simulink library "halin"  (R2021b)
settings: Solver=VariableStepAuto  StartTime=0.0  StopTime=10.0  RelTol=1e-3
undefined symbols (not defined in the file): KHAL_CAN1ABM1E2E_flg, KHAL_CAN1ESC1E2E_flg, KHAL_CAN1ESC5E2E_flg, KHAL_CAN1ESC7E2E_flg, KHAL_CAN1FCM2E2E_flg, KHAL_CAN1FCM3E2E_flg, KHAL_CAN1FCM4E2E_flg, KHAL_CAN3BMS1E2E_flg, KHAL_CAN3BMS6E2E_flg, KHAL_CAN3CCU1E2E_flg, KHAL_CAN3CCU2E2E_flg, KHAL_CAN3MCUF1E2E_flg, KHAL_CAN3MCUR1E2E_flg, KHAL_CAN3Shifter1E2E_flg, TRUE
libraries: simulink x420, FVT_lib x149, hcu_lib x49
(part 8 of 14)

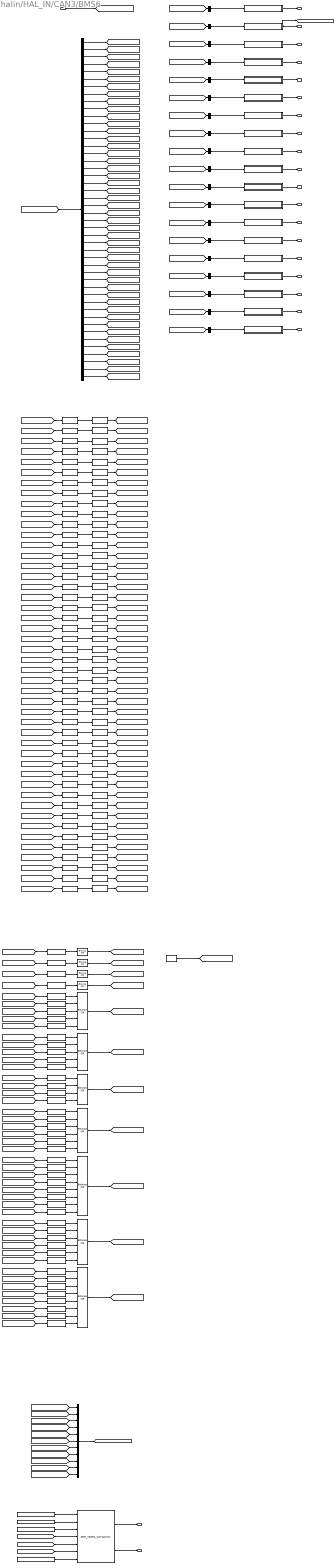
== system halin/HAL_IN/CAN3/BMS6 ==
  DT_CAN3_SG_BMS6 : Inport
  0x3b : Constant  Value=0x3b
  0xdb : Constant  Value=0xdb
  BMSChckSum : Subsystem
  BMSREADY : Subsystem
  BMSRolCnct : Subsystem
  BMSWarn1 : Subsystem
  BMSWarn2 : Subsystem
  BMSWarn3 : Subsystem
  BMSWarn4 : Subsystem
  BMSWarn5 : Subsystem
  BMSWarn6 : Subsystem
  BMSWarn7 : Subsystem
  BMSWarn8 : Subsystem
  BitwiseAND{,1..45} (46 alike) : simulink/Logic and Bit Operations/Bitwise Operator  logicop=AND  UseBitMask=on  BitMask=0xFF  BitMaskRealWorld=Stored Integer
  BitwiseOR{,1..3} (4 alike) : simulink/Logic and Bit Operations/Bitwise Operator  logicop=OR  UseBitMask=off  BitMask=bin2dec('11011001')  BitMaskRealWorld=Stored Integer
  BitwiseOR10 : simulink/Logic and Bit Operations/Bitwise Operator  logicop=OR  UseBitMask=off  NumInputPorts=8  BitMask=bin2dec('11011001')  BitMaskRealWorld=Stored Integer
  BitwiseOR4 : simulink/Logic and Bit Operations/Bitwise Operator  logicop=OR  UseBitMask=off  NumInputPorts=5  BitMask=bin2dec('11011001')  BitMaskRealWorld=Stored Integer
  BitwiseOR5 : simulink/Logic and Bit Operations/Bitwise Operator  logicop=OR  UseBitMask=off  NumInputPorts=5  BitMask=bin2dec('11011001')  BitMaskRealWorld=Stored Integer
  BitwiseOR6 : simulink/Logic and Bit Operations/Bitwise Operator  logicop=OR  UseBitMask=off  NumInputPorts=4  BitMask=bin2dec('11011001')  BitMaskRealWorld=Stored Integer
  BitwiseOR7 : simulink/Logic and Bit Operations/Bitwise Operator  logicop=OR  UseBitMask=off  NumInputPorts=6  BitMask=bin2dec('11011001')  BitMaskRealWorld=Stored Integer
  BitwiseOR8 : simulink/Logic and Bit Operations/Bitwise Operator  logicop=OR  UseBitMask=off  NumInputPorts=8  BitMask=bin2dec('11011001')  BitMaskRealWorld=Stored Integer
  BitwiseOR9 : simulink/Logic and Bit Operations/Bitwise Operator  logicop=OR  UseBitMask=off  NumInputPorts=6  BitMask=bin2dec('11011001')  BitMaskRealWorld=Stored Integer
  ChrgPlugSta : Subsystem
  DDM_CS&RC_Comparison : FVT_lib/hal/DDM_CS&RC_Comparison  MsgCycleTime=100
  Data Type Conversion{,1..45} (46 alike) : DataTypeConversion  OutDataTypeStr=uint8
  ExtChrgSta : Subsystem
  HVBContactorSta : Subsystem
  HVBHVILErr : Subsystem
  HVBPreheatPrecoolSta : Subsystem
  HVBattReady4Pre : Subsystem
  HVILSta : Subsystem
  KHAL_CAN3BMS6E2E_flg : Constant  Value=KHAL_CAN3BMS6E2E_flg
  LeftShift{,3,14,17,22,25,29,41,43,45} (10 alike) : ArithShift  BitShiftDirection=Left
  LeftShift{1,7,12,16,18,27,30..31} (8 alike) : ArithShift  BitShiftNumber=4  BitShiftDirection=Left
  LeftShift{10,24,35,42} (4 alike) : ArithShift  BitShiftNumber=7  BitShiftDirection=Left
  LeftShift{5,11,13,20,23,28,39} (7 alike) : ArithShift  BitShiftNumber=2  BitShiftDirection=Left
  LeftShift{9,15,19,32..34,36} (7 alike) : ArithShift  BitShiftNumber=6  BitShiftDirection=Left
  LeftShift{2,4,21,26,44} (5 alike) : ArithShift  BitShiftNumber=1  BitShiftDirection=Left
  LeftShift37 : ArithShift  BitShiftNumber=5  BitShiftDirection=Left
  LeftShift38 : ArithShift  BitShiftNumber=3  BitShiftDirection=Left
  LeftShift40 : ArithShift  BitShiftNumber=5  BitShiftDirection=Left
  LeftShift6 : ArithShift  BitShiftNumber=3  BitShiftDirection=Left
  LeftShift8 : ArithShift  BitShiftNumber=5  BitShiftDirection=Left
  MessageRollingCounter : FVT_lib/hal/MessageRollingCounter  CounterMAX=14  task_time_ms=5  msg_time_ms=100
  Mux : Mux  Inputs=11
  V2LSta : Subsystem
  bus_selector : BusSelector  OutputSignals=CAN3_BMSChckSum,CAN3_BMSRolCnct,CAN3_BMS_READY,CAN3_BMS_Warn_1,CAN3_BMS_Warn_2,CAN3_BMS_Warn_3,CAN3_BMS_Warn_4,CAN3_BMS_Warn_5,CAN3_BMS_Warn_6,CAN3_BMS_Warn_7,CAN3_BMS_Warn_8,CAN3_CellUnconsistErr,CAN3_ChrgInLockReq,CAN3_ChrgPlugSta,CAN3_DCChrgSysShockErr,CAN3_DisChrgPlugErr,CAN3_ExtChrgSta,CAN3_HVBCellOvrVoltErr,CAN3_HVBCellOvrVoltWarn,CAN3_HVBCellUdrVoltWarn,CAN3_HVBCellUnbalanErr,CAN3_HVBCellUndrVoltErr,CAN3_HVBChrgErr,CAN3_HVBContactorSta,CAN3_HVBHVILErr,CAN3_HVBOvrChrgCurrErr,CAN3_HVBOvrDchrgCurErr,CAN3_HVBOvrSOCErr,CAN3_HVBOvrTempErr,CAN3_HVBOvrTempWarn,CAN3_HVBOvrVoltErr,CAN3_HVBPrechrgSta,CAN3_HVBPreheatPrecoolSta,CAN3_HVBSOCJumpError,CAN3_HVBShrtChrgCurrErr,CAN3_HVBShrtDischrgCurrErr,CAN3_HVBTempDiffErr,CAN3_HVBUndrSOCErr,CAN3_HVBUndrTempErr,CAN3_HVBUndrTempWarn,CAN3_HVBUndrVoltErr,CAN3_HVBattReady4Pre,CAN3_HVILSta,CAN3_IsoDetSta,CAN3_SystemUncomErr,CAN3_V2LSta
  bus_selector1 : BusSelector  OutputSignals=CAN3_BMSChckSum
  bus_selector10 : BusSelector  OutputSignals=CAN3_BMS_Warn_7
  bus_selector11 : BusSelector  OutputSignals=CAN3_BMS_Warn_8
  bus_selector12 : BusSelector  OutputSignals=CAN3_ChrgPlugSta
  bus_selector13 : BusSelector  OutputSignals=CAN3_ExtChrgSta
  bus_selector14 : BusSelector  OutputSignals=CAN3_HVBContactorSta
  bus_selector15 : BusSelector  OutputSignals=CAN3_HVBHVILErr
  bus_selector16 : BusSelector  OutputSignals=CAN3_HVBPreheatPrecoolSta
  bus_selector17 : BusSelector  OutputSignals=CAN3_HVBattReady4Pre
  bus_selector18 : BusSelector  OutputSignals=CAN3_HVILSta
  bus_selector19 : BusSelector  OutputSignals=CAN3_V2LSta
  bus_selector2 : BusSelector  OutputSignals=CAN3_BMSRolCnct
  bus_selector3 : BusSelector  OutputSignals=CAN3_BMS_READY
  bus_selector4 : BusSelector  OutputSignals=CAN3_BMS_Warn_1
  bus_selector5 : BusSelector  OutputSignals=CAN3_BMS_Warn_2
  bus_selector6 : BusSelector  OutputSignals=CAN3_BMS_Warn_3
  bus_selector7 : BusSelector  OutputSignals=CAN3_BMS_Warn_4
  bus_selector8 : BusSelector  OutputSignals=CAN3_BMS_Warn_5
  bus_selector9 : BusSelector  OutputSignals=CAN3_BMS_Warn_6
  constant : Constant  Value=0x0  OutDataTypeStr=uint8
  VHAL_BMS6CSErr_flg : Outport
  VHAL_BMS6RCErr_flg : Outport  Port=2
  VHAL_BMSChckSum_enum : Outport  Port=3
  VHAL_BMSRolCnct_enum : Outport  Port=4
  VHAL_BMSREADY_flg : Outport  Port=5
  VHAL_BMSWarn1_flg : Outport  Port=6
  VHAL_BMSWarn2_flg : Outport  Port=7
  VHAL_BMSWarn3_flg : Outport  Port=8
  VHAL_BMSWarn4_flg : Outport  Port=9
  VHAL_BMSWarn5_flg : Outport  Port=10
  VHAL_BMSWarn6_flg : Outport  Port=11
  VHAL_BMSWarn7_flg : Outport  Port=12
  VHAL_BMSWarn8_flg : Outport  Port=13
  VHAL_ChrgPlugSta_enum : Outport  Port=14
  VHAL_ExtChrgSta_enum : Outport  Port=15
  VHAL_HVBContactorSta_flg : Outport  Port=16
  VHAL_HVBHVILErr_flg : Outport  Port=17
  VHAL_HVBPreheatPrecoolSta_enum : Outport  Port=18
  VHAL_HVBattReady4Pre_enum : Outport  Port=19
  VHAL_HVILSta_flg : Outport  Port=20
  VHAL_V2LSta_enum : Outport  Port=21
  wires:
  DT_CAN3_SG_BMS6/1 -> [DT_CAN3_SG_BMS6]
  [DT_CAN3_SG_BMS6] -> bus_selector/1
  bus_selector/1 -> [CAN3_BMSChckSum]  "<CAN3_BMSChckSum>"
  [CAN3_BMSChckSum] -> LeftShift/1
  LeftShift/1 -> BitwiseAND/1
  BitwiseAND/1 -> [Byte_0_CAN3_BMSChckSum]
  bus_selector/2 -> [CAN3_BMSRolCnct]  "<CAN3_BMSRolCnct>"
  [CAN3_BMSRolCnct] -> LeftShift1/1
  LeftShift1/1 -> BitwiseAND1/1
  BitwiseAND1/1 -> [Byte_1_CAN3_BMSRolCnct]
  bus_selector/3 -> [CAN3_BMS_READY]  "<CAN3_BMS_READY>"
  [CAN3_BMS_READY] -> LeftShift2/1
  LeftShift2/1 -> BitwiseAND2/1
  BitwiseAND2/1 -> [Byte_8_CAN3_BMS_READY]
  bus_selector/4 -> [CAN3_BMS_Warn_1]  "<CAN3_BMS_Warn_1>"
  [CAN3_BMS_Warn_1] -> LeftShift3/1
  LeftShift3/1 -> BitwiseAND3/1
  BitwiseAND3/1 -> [Byte_11_CAN3_BMS_Warn_1]
  bus_selector/5 -> [CAN3_BMS_Warn_2]  "<CAN3_BMS_Warn_2>"
  [CAN3_BMS_Warn_2] -> LeftShift4/1
  LeftShift4/1 -> BitwiseAND4/1
  BitwiseAND4/1 -> [Byte_11_CAN3_BMS_Warn_2]
  bus_selector/6 -> [CAN3_BMS_Warn_3]  "<CAN3_BMS_Warn_3>"
  [CAN3_BMS_Warn_3] -> LeftShift5/1
  LeftShift5/1 -> BitwiseAND5/1
  BitwiseAND5/1 -> [Byte_11_CAN3_BMS_Warn_3]
  bus_selector/7 -> [CAN3_BMS_Warn_4]  "<CAN3_BMS_Warn_4>"
  [CAN3_BMS_Warn_4] -> LeftShift6/1
  LeftShift6/1 -> BitwiseAND6/1
  BitwiseAND6/1 -> [Byte_11_CAN3_BMS_Warn_4]
  bus_selector/8 -> [CAN3_BMS_Warn_5]  "<CAN3_BMS_Warn_5>"
  [CAN3_BMS_Warn_5] -> LeftShift7/1
  LeftShift7/1 -> BitwiseAND7/1
  BitwiseAND7/1 -> [Byte_11_CAN3_BMS_Warn_5]
  bus_selector/9 -> [CAN3_BMS_Warn_6]  "<CAN3_BMS_Warn_6>"
  [CAN3_BMS_Warn_6] -> LeftShift8/1
  LeftShift8/1 -> BitwiseAND8/1
  BitwiseAND8/1 -> [Byte_11_CAN3_BMS_Warn_6]
  bus_selector/10 -> [CAN3_BMS_Warn_7]  "<CAN3_BMS_Warn_7>"
  [CAN3_BMS_Warn_7] -> LeftShift9/1
  LeftShift9/1 -> BitwiseAND9/1
  BitwiseAND9/1 -> [Byte_11_CAN3_BMS_Warn_7]
  bus_selector/11 -> [CAN3_BMS_Warn_8]  "<CAN3_BMS_Warn_8>"
  [CAN3_BMS_Warn_8] -> LeftShift10/1
  LeftShift10/1 -> BitwiseAND10/1
  BitwiseAND10/1 -> [Byte_11_CAN3_BMS_Warn_8]
  bus_selector/12 -> [CAN3_CellUnconsistErr]  "<CAN3_CellUnconsistErr>"
  [CAN3_CellUnconsistErr] -> LeftShift11/1
  LeftShift11/1 -> BitwiseAND11/1
  BitwiseAND11/1 -> [Byte_6_CAN3_CellUnconsistErr]
  bus_selector/13 -> [CAN3_ChrgInLockReq]  "<CAN3_ChrgInLockReq>"
  [CAN3_ChrgInLockReq] -> LeftShift12/1
  LeftShift12/1 -> BitwiseAND12/1
  BitwiseAND12/1 -> [Byte_5_CAN3_ChrgInLockReq]
  bus_selector/14 -> [CAN3_ChrgPlugSta]  "<CAN3_ChrgPlugSta>"
  [CAN3_ChrgPlugSta] -> LeftShift13/1
  LeftShift13/1 -> BitwiseAND13/1
  BitwiseAND13/1 -> [Byte_7_CAN3_ChrgPlugSta]
  bus_selector/15 -> [CAN3_DCChrgSysShockErr]  "<CAN3_DCChrgSysShockErr>"
  [CAN3_DCChrgSysShockErr] -> LeftShift14/1
  LeftShift14/1 -> BitwiseAND14/1
  BitwiseAND14/1 -> [Byte_8_CAN3_DCChrgSysShockErr]
  bus_selector/16 -> [CAN3_DisChrgPlugErr]  "<CAN3_DisChrgPlugErr>"
  [CAN3_DisChrgPlugErr] -> LeftShift15/1
  LeftShift15/1 -> BitwiseAND15/1
  BitwiseAND15/1 -> [Byte_5_CAN3_DisChrgPlugErr]
  bus_selector/17 -> [CAN3_ExtChrgSta]  "<CAN3_ExtChrgSta>"
  [CAN3_ExtChrgSta] -> LeftShift16/1
  LeftShift16/1 -> BitwiseAND16/1
  BitwiseAND16/1 -> [Byte_7_CAN3_ExtChrgSta]
  bus_selector/18 -> [CAN3_HVBCellOvrVoltErr]  "<CAN3_HVBCellOvrVoltErr>"
  [CAN3_HVBCellOvrVoltErr] -> LeftShift17/1
  LeftShift17/1 -> BitwiseAND17/1
  BitwiseAND17/1 -> [Byte_5_CAN3_HVBCellOvrVoltErr]
  bus_selector/19 -> [CAN3_HVBCellOvrVoltWarn]  "<CAN3_HVBCellOvrVoltWarn>"
  [CAN3_HVBCellOvrVoltWarn] -> LeftShift18/1
  LeftShift18/1 -> BitwiseAND18/1
  BitwiseAND18/1 -> [Byte_6_CAN3_HVBCellOvrVoltWarn]
  bus_selector/20 -> [CAN3_HVBCellUdrVoltWarn]  "<CAN3_HVBCellUdrVoltWarn>"
  [CAN3_HVBCellUdrVoltWarn] -> LeftShift19/1
  LeftShift19/1 -> BitwiseAND19/1
  BitwiseAND19/1 -> [Byte_6_CAN3_HVBCellUdrVoltWarn]
  bus_selector/21 -> [CAN3_HVBCellUnbalanErr]  "<CAN3_HVBCellUnbalanErr>"
  [CAN3_HVBCellUnbalanErr] -> LeftShift20/1
  LeftShift20/1 -> BitwiseAND20/1
  BitwiseAND20/1 -> [Byte_5_CAN3_HVBCellUnbalanErr]
  bus_selector/22 -> [CAN3_HVBCellUndrVoltErr]  "<CAN3_HVBCellUndrVoltErr>"
  [CAN3_HVBCellUndrVoltErr] -> LeftShift21/1
  LeftShift21/1 -> BitwiseAND21/1
  BitwiseAND21/1 -> [Byte_5_CAN3_HVBCellUndrVoltErr]
  bus_selector/23 -> [CAN3_HVBChrgErr]  "<CAN3_HVBChrgErr>"
  [CAN3_HVBChrgErr] -> LeftShift22/1
  LeftShift22/1 -> BitwiseAND22/1
  BitwiseAND22/1 -> [Byte_4_CAN3_HVBChrgErr]
  bus_selector/24 -> [CAN3_HVBContactorSta]  "<CAN3_HVBContactorSta>"
  [CAN3_HVBContactorSta] -> LeftShift23/1
  LeftShift23/1 -> BitwiseAND23/1
  BitwiseAND23/1 -> [Byte_8_CAN3_HVBContactorSta]
  bus_selector/25 -> [CAN3_HVBHVILErr]  "<CAN3_HVBHVILErr>"
  [CAN3_HVBHVILErr] -> LeftShift24/1
  LeftShift24/1 -> BitwiseAND24/1
  BitwiseAND24/1 -> [Byte_9_CAN3_HVBHVILErr]
  bus_selector/26 -> [CAN3_HVBOvrChrgCurrErr]  "<CAN3_HVBOvrChrgCurrErr>"
  [CAN3_HVBOvrChrgCurrErr] -> LeftShift25/1
  LeftShift25/1 -> BitwiseAND25/1
  BitwiseAND25/1 -> [Byte_9_CAN3_HVBOvrChrgCurrErr]
  bus_selector/27 -> [CAN3_HVBOvrDchrgCurErr]  "<CAN3_HVBOvrDchrgCurErr>"
  [CAN3_HVBOvrDchrgCurErr] -> LeftShift26/1
  LeftShift26/1 -> BitwiseAND26/1
  BitwiseAND26/1 -> [Byte_9_CAN3_HVBOvrDchrgCurErr]
  bus_selector/28 -> [CAN3_HVBOvrSOCErr]  "<CAN3_HVBOvrSOCErr>"
  [CAN3_HVBOvrSOCErr] -> LeftShift27/1
  LeftShift27/1 -> BitwiseAND27/1
  BitwiseAND27/1 -> [Byte_9_CAN3_HVBOvrSOCErr]
  bus_selector/29 -> [CAN3_HVBOvrTempErr]  "<CAN3_HVBOvrTempErr>"
  [CAN3_HVBOvrTempErr] -> LeftShift28/1
  LeftShift28/1 -> BitwiseAND28/1
  BitwiseAND28/1 -> [Byte_9_CAN3_HVBOvrTempErr]
  bus_selector/30 -> [CAN3_HVBOvrTempWarn]  "<CAN3_HVBOvrTempWarn>"
  [CAN3_HVBOvrTempWarn] -> LeftShift29/1
  LeftShift29/1 -> BitwiseAND29/1
  BitwiseAND29/1 -> [Byte_10_CAN3_HVBOvrTempWarn]
  bus_selector/31 -> [CAN3_HVBOvrVoltErr]  "<CAN3_HVBOvrVoltErr>"
  [CAN3_HVBOvrVoltErr] -> LeftShift30/1
  LeftShift30/1 -> BitwiseAND30/1
  BitwiseAND30/1 -> [Byte_10_CAN3_HVBOvrVoltErr]
  bus_selector/32 -> [CAN3_HVBPrechrgSta]  "<CAN3_HVBPrechrgSta>"
  [CAN3_HVBPrechrgSta] -> LeftShift31/1
  LeftShift31/1 -> BitwiseAND31/1
  BitwiseAND31/1 -> [Byte_8_CAN3_HVBPrechrgSta]
  bus_selector/33 -> [CAN3_HVBPreheatPrecoolSta]  "<CAN3_HVBPreheatPrecoolSta>"
  [CAN3_HVBPreheatPrecoolSta] -> LeftShift32/1
  LeftShift32/1 -> BitwiseAND32/1
  BitwiseAND32/1 -> [Byte_7_CAN3_HVBPreheatPrecoolSta]
  bus_selector/34 -> [CAN3_HVBSOCJumpError]  "<CAN3_HVBSOCJumpError>"
  [CAN3_HVBSOCJumpError] -> LeftShift33/1
  LeftShift33/1 -> BitwiseAND33/1
  BitwiseAND33/1 -> [Byte_9_CAN3_HVBSOCJumpError]
  bus_selector/35 -> [CAN3_HVBShrtChrgCurrErr]  "<CAN3_HVBShrtChrgCurrErr>"
  [CAN3_HVBShrtChrgCurrErr] -> LeftShift34/1
  LeftShift34/1 -> BitwiseAND34/1
  BitwiseAND34/1 -> [Byte_10_CAN3_HVBShrtChrgCurrErr]
  bus_selector/36 -> [CAN3_HVBShrtDischrgCurrErr]  "<CAN3_HVBShrtDischrgCurrErr>"
  [CAN3_HVBShrtDischrgCurrErr] -> LeftShift35/1
  LeftShift35/1 -> BitwiseAND35/1
  BitwiseAND35/1 -> [Byte_10_CAN3_HVBShrtDischrgCurrErr]
  bus_selector/37 -> [CAN3_HVBTempDiffErr]  "<CAN3_HVBTempDiffErr>"
  [CAN3_HVBTempDiffErr] -> LeftShift36/1
  LeftShift36/1 -> BitwiseAND36/1
  BitwiseAND36/1 -> [Byte_8_CAN3_HVBTempDiffErr]
  bus_selector/38 -> [CAN3_HVBUndrSOCErr]  "<CAN3_HVBUndrSOCErr>"
  [CAN3_HVBUndrSOCErr] -> LeftShift37/1
  LeftShift37/1 -> BitwiseAND37/1
  BitwiseAND37/1 -> [Byte_9_CAN3_HVBUndrSOCErr]
  bus_selector/39 -> [CAN3_HVBUndrTempErr]  "<CAN3_HVBUndrTempErr>"
  [CAN3_HVBUndrTempErr] -> LeftShift38/1
  LeftShift38/1 -> BitwiseAND38/1
  BitwiseAND38/1 -> [Byte_9_CAN3_HVBUndrTempErr]
  bus_selector/40 -> [CAN3_HVBUndrTempWarn]  "<CAN3_HVBUndrTempWarn>"
  [CAN3_HVBUndrTempWarn] -> LeftShift39/1
  LeftShift39/1 -> BitwiseAND39/1
  BitwiseAND39/1 -> [Byte_10_CAN3_HVBUndrTempWarn]
  bus_selector/41 -> [CAN3_HVBUndrVoltErr]  "<CAN3_HVBUndrVoltErr>"
  [CAN3_HVBUndrVoltErr] -> LeftShift40/1
  LeftShift40/1 -> BitwiseAND40/1
  BitwiseAND40/1 -> [Byte_10_CAN3_HVBUndrVoltErr]
  bus_selector/42 -> [CAN3_HVBattReady4Pre]  "<CAN3_HVBattReady4Pre>"
  [CAN3_HVBattReady4Pre] -> LeftShift41/1
  LeftShift41/1 -> BitwiseAND41/1
  BitwiseAND41/1 -> [Byte_7_CAN3_HVBattReady4Pre]
  bus_selector/43 -> [CAN3_HVILSta]  "<CAN3_HVILSta>"
  [CAN3_HVILSta] -> LeftShift42/1
  LeftShift42/1 -> BitwiseAND42/1
  BitwiseAND42/1 -> [Byte_8_CAN3_HVILSta]
  bus_selector/44 -> [CAN3_IsoDetSta]  "<CAN3_IsoDetSta>"
  [CAN3_IsoDetSta] -> LeftShift43/1
  LeftShift43/1 -> BitwiseAND43/1
  BitwiseAND43/1 -> [Byte_6_CAN3_IsoDetSta]
  bus_selector/45 -> [CAN3_SystemUncomErr]  "<CAN3_SystemUncomErr>"
  [CAN3_SystemUncomErr] -> LeftShift44/1
  LeftShift44/1 -> BitwiseAND44/1
  BitwiseAND44/1 -> [Byte_6_CAN3_SystemUncomErr]
  bus_selector/46 -> [CAN3_V2LSta]  "<CAN3_V2LSta>"
  [CAN3_V2LSta] -> LeftShift45/1
  LeftShift45/1 -> BitwiseAND45/1
  BitwiseAND45/1 -> [Byte_3_CAN3_V2LSta]
  Data Type Conversion/1 -> BitwiseOR/1
  [Byte_0_CAN3_BMSChckSum] -> Data Type Conversion/1
  BitwiseOR/1 -> [Byte_0]
  Data Type Conversion1/1 -> BitwiseOR1/1
  [Byte_1_CAN3_BMSRolCnct] -> Data Type Conversion1/1
  BitwiseOR1/1 -> [Byte_1]
  constant/1 -> [Byte_2]
  Data Type Conversion2/1 -> BitwiseOR2/1
  [Byte_3_CAN3_V2LSta] -> Data Type Conversion2/1
  BitwiseOR2/1 -> [Byte_3]
  Data Type Conversion3/1 -> BitwiseOR3/1
  [Byte_4_CAN3_HVBChrgErr] -> Data Type Conversion3/1
  BitwiseOR3/1 -> [Byte_4]
  Data Type Conversion4/1 -> BitwiseOR4/1
  [Byte_5_CAN3_ChrgInLockReq] -> Data Type Conversion4/1
  Data Type Conversion5/1 -> BitwiseOR4/2
  [Byte_5_CAN3_DisChrgPlugErr] -> Data Type Conversion5/1
  Data Type Conversion6/1 -> BitwiseOR4/3
  [Byte_5_CAN3_HVBCellOvrVoltErr] -> Data Type Conversion6/1
  Data Type Conversion7/1 -> BitwiseOR4/4
  [Byte_5_CAN3_HVBCellUnbalanErr] -> Data Type Conversion7/1
  Data Type Conversion8/1 -> BitwiseOR4/5
  [Byte_5_CAN3_HVBCellUndrVoltErr] -> Data Type Conversion8/1
  BitwiseOR4/1 -> [Byte_5]
  Data Type Conversion9/1 -> BitwiseOR5/1
  [Byte_6_CAN3_CellUnconsistErr] -> Data Type Conversion9/1
  Data Type Conversion10/1 -> BitwiseOR5/2
  [Byte_6_CAN3_HVBCellOvrVoltWarn] -> Data Type Conversion10/1
  Data Type Conversion11/1 -> BitwiseOR5/3
  [Byte_6_CAN3_HVBCellUdrVoltWarn] -> Data Type Conversion11/1
  Data Type Conversion12/1 -> BitwiseOR5/4
  [Byte_6_CAN3_IsoDetSta] -> Data Type Conversion12/1
  Data Type Conversion13/1 -> BitwiseOR5/5
  [Byte_6_CAN3_SystemUncomErr] -> Data Type Conversion13/1
  BitwiseOR5/1 -> [Byte_6]
  Data Type Conversion14/1 -> BitwiseOR6/1
  [Byte_7_CAN3_ChrgPlugSta] -> Data Type Conversion14/1
  Data Type Conversion15/1 -> BitwiseOR6/2
  [Byte_7_CAN3_ExtChrgSta] -> Data Type Conversion15/1
  Data Type Conversion16/1 -> BitwiseOR6/3
  [Byte_7_CAN3_HVBPreheatPrecoolSta] -> Data Type Conversion16/1
  Data Type Conversion17/1 -> BitwiseOR6/4
  [Byte_7_CAN3_HVBattReady4Pre] -> Data Type Conversion17/1
  BitwiseOR6/1 -> [Byte_7]
  Data Type Conversion18/1 -> BitwiseOR7/1
  [Byte_8_CAN3_BMS_READY] -> Data Type Conversion18/1
  Data Type Conversion19/1 -> BitwiseOR7/2
  [Byte_8_CAN3_DCChrgSysShockErr] -> Data Type Conversion19/1
  Data Type Conversion20/1 -> BitwiseOR7/3
  [Byte_8_CAN3_HVBContactorSta] -> Data Type Conversion20/1
  Data Type Conversion21/1 -> BitwiseOR7/4
  [Byte_8_CAN3_HVBPrechrgSta] -> Data Type Conversion21/1
  Data Type Conversion22/1 -> BitwiseOR7/5
  [Byte_8_CAN3_HVBTempDiffErr] -> Data Type Conversion22/1
  Data Type Conversion23/1 -> BitwiseOR7/6
  [Byte_8_CAN3_HVILSta] -> Data Type Conversion23/1
  BitwiseOR7/1 -> [Byte_8]
  Data Type Conversion24/1 -> BitwiseOR8/1
  [Byte_9_CAN3_HVBHVILErr] -> Data Type Conversion24/1
  Data Type Conversion25/1 -> BitwiseOR8/2
  [Byte_9_CAN3_HVBOvrChrgCurrErr] -> Data Type Conversion25/1
  Data Type Conversion26/1 -> BitwiseOR8/3
  [Byte_9_CAN3_HVBOvrDchrgCurErr] -> Data Type Conversion26/1
  Data Type Conversion27/1 -> BitwiseOR8/4
  [Byte_9_CAN3_HVBOvrSOCErr] -> Data Type Conversion27/1
  Data Type Conversion28/1 -> BitwiseOR8/5
  [Byte_9_CAN3_HVBOvrTempErr] -> Data Type Conversion28/1
  Data Type Conversion29/1 -> BitwiseOR8/6
  [Byte_9_CAN3_HVBSOCJumpError] -> Data Type Conversion29/1
  Data Type Conversion30/1 -> BitwiseOR8/7
  [Byte_9_CAN3_HVBUndrSOCErr] -> Data Type Conversion30/1
  Data Type Conversion31/1 -> BitwiseOR8/8
  [Byte_9_CAN3_HVBUndrTempErr] -> Data Type Conversion31/1
  BitwiseOR8/1 -> [Byte_9]
  Data Type Conversion32/1 -> BitwiseOR9/1
  [Byte_10_CAN3_HVBOvrTempWarn] -> Data Type Conversion32/1
  Data Type Conversion33/1 -> BitwiseOR9/2
  [Byte_10_CAN3_HVBOvrVoltErr] -> Data Type Conversion33/1
  Data Type Conversion34/1 -> BitwiseOR9/3
  [Byte_10_CAN3_HVBShrtChrgCurrErr] -> Data Type Conversion34/1
  Data Type Conversion35/1 -> BitwiseOR9/4
  [Byte_10_CAN3_HVBShrtDischrgCurrErr] -> Data Type Conversion35/1
  Data Type Conversion36/1 -> BitwiseOR9/5
  [Byte_10_CAN3_HVBUndrTempWarn] -> Data Type Conversion36/1
  Data Type Conversion37/1 -> BitwiseOR9/6
  [Byte_10_CAN3_HVBUndrVoltErr] -> Data Type Conversion37/1
  BitwiseOR9/1 -> [Byte_10]
  Data Type Conversion38/1 -> BitwiseOR10/1
  [Byte_11_CAN3_BMS_Warn_1] -> Data Type Conversion38/1
  Data Type Conversion39/1 -> BitwiseOR10/2
  [Byte_11_CAN3_BMS_Warn_2] -> Data Type Conversion39/1
  Data Type Conversion40/1 -> BitwiseOR10/3
  [Byte_11_CAN3_BMS_Warn_3] -> Data Type Conversion40/1
  Data Type Conversion41/1 -> BitwiseOR10/4
  [Byte_11_CAN3_BMS_Warn_4] -> Data Type Conversion41/1
  Data Type Conversion42/1 -> BitwiseOR10/5
  [Byte_11_CAN3_BMS_Warn_5] -> Data Type Conversion42/1
  Data Type Conversion43/1 -> BitwiseOR10/6
  [Byte_11_CAN3_BMS_Warn_6] -> Data Type Conversion43/1
  Data Type Conversion44/1 -> BitwiseOR10/7
  [Byte_11_CAN3_BMS_Warn_7] -> Data Type Conversion44/1
  Data Type Conversion45/1 -> BitwiseOR10/8
  [Byte_11_CAN3_BMS_Warn_8] -> Data Type Conversion45/1
  BitwiseOR10/1 -> [Byte_11]
  [Byte_1] -> Mux/1
  [Byte_2] -> Mux/2
  [Byte_3] -> Mux/3
  [Byte_4] -> Mux/4
  [Byte_5] -> Mux/5
  [Byte_6] -> Mux/6
  [Byte_7] -> Mux/7
  [Byte_8] -> Mux/8
  [Byte_9] -> Mux/9
  [Byte_10] -> Mux/10
  [Byte_11] -> Mux/11
  Mux/1 -> [VHAL_CAN3BMS6noCS_raw]
  KHAL_CAN3BMS6E2E_flg/1 -> DDM_CS&RC_Comparison/1
  0x3b/1 -> DDM_CS&RC_Comparison/2
  0xdb/1 -> DDM_CS&RC_Comparison/3
  [VHAL_CAN3BMS6noCS_raw] -> DDM_CS&RC_Comparison/4
  [Byte_0] -> DDM_CS&RC_Comparison/5
  [RC_ECU] -> DDM_CS&RC_Comparison/6
  MessageRollingCounter/1 -> DDM_CS&RC_Comparison/7
  DDM_CS&RC_Comparison/1 -> VHAL_BMS6CSErr_flg/1
  DDM_CS&RC_Comparison/2 -> VHAL_BMS6RCErr_flg/1
  [DT_CAN3_SG_BMS6] -> bus_selector1/1
  bus_selector1/1 -> BMSChckSum/1(BMSChckSum)  "<CAN3_BMSChckSum>"
  BMSChckSum/1(VHAL_BMSChckSum_enum) -> VHAL_BMSChckSum_enum/1
  [DT_CAN3_SG_BMS6] -> bus_selector2/1
  bus_selector2/1 -> BMSRolCnct/1(BMSRolCnct)  "<CAN3_BMSRolCnct>"
  BMSRolCnct/1(VHAL_BMSRolCnct_enum) -> VHAL_BMSRolCnct_enum/1, [RC_ECU]
  [DT_CAN3_SG_BMS6] -> bus_selector3/1
  bus_selector3/1 -> BMSREADY/1(BMS_READY)  "<CAN3_BMS_READY>"
  BMSREADY/1(VHAL_BMSREADY_flg) -> VHAL_BMSREADY_flg/1
  [DT_CAN3_SG_BMS6] -> bus_selector4/1
  bus_selector4/1 -> BMSWarn1/1(BMS_Warn_1)  "<CAN3_BMS_Warn_1>"
  BMSWarn1/1(VHAL_BMSWarn1_flg) -> VHAL_BMSWarn1_flg/1
  [DT_CAN3_SG_BMS6] -> bus_selector5/1
  bus_selector5/1 -> BMSWarn2/1(BMS_Warn_2)  "<CAN3_BMS_Warn_2>"
  BMSWarn2/1(VHAL_BMSWarn2_flg) -> VHAL_BMSWarn2_flg/1
  [DT_CAN3_SG_BMS6] -> bus_selector6/1
  bus_selector6/1 -> BMSWarn3/1(BMS_Warn_3)  "<CAN3_BMS_Warn_3>"
  BMSWarn3/1(VHAL_BMSWarn3_flg) -> VHAL_BMSWarn3_flg/1
  [DT_CAN3_SG_BMS6] -> bus_selector7/1
  bus_selector7/1 -> BMSWarn4/1(BMS_Warn_4)  "<CAN3_BMS_Warn_4>"
  BMSWarn4/1(VHAL_BMSWarn4_flg) -> VHAL_BMSWarn4_flg/1
  [DT_CAN3_SG_BMS6] -> bus_selector8/1
  bus_selector8/1 -> BMSWarn5/1(BMS_Warn_5)  "<CAN3_BMS_Warn_5>"
  BMSWarn5/1(VHAL_BMSWarn5_flg) -> VHAL_BMSWarn5_flg/1
  [DT_CAN3_SG_BMS6] -> bus_selector9/1
  bus_selector9/1 -> BMSWarn6/1(BMS_Warn_6)  "<CAN3_BMS_Warn_6>"
  BMSWarn6/1(VHAL_BMSWarn6_flg) -> VHAL_BMSWarn6_flg/1
  [DT_CAN3_SG_BMS6] -> bus_selector10/1
  bus_selector10/1 -> BMSWarn7/1(BMS_Warn_7)  "<CAN3_BMS_Warn_7>"
  BMSWarn7/1(VHAL_BMSWarn7_flg) -> VHAL_BMSWarn7_flg/1
  [DT_CAN3_SG_BMS6] -> bus_selector11/1
  bus_selector11/1 -> BMSWarn8/1(BMS_Warn_8)  "<CAN3_BMS_Warn_8>"
  BMSWarn8/1(VHAL_BMSWarn8_flg) -> VHAL_BMSWarn8_flg/1
  [DT_CAN3_SG_BMS6] -> bus_selector12/1
  bus_selector12/1 -> ChrgPlugSta/1(ChrgPlugSta)  "<CAN3_ChrgPlugSta>"
  ChrgPlugSta/1(VHAL_ChrgPlugSta_enum) -> VHAL_ChrgPlugSta_enum/1
  [DT_CAN3_SG_BMS6] -> bus_selector13/1
  bus_selector13/1 -> ExtChrgSta/1(ExtChrgSta)  "<CAN3_ExtChrgSta>"
  ExtChrgSta/1(VHAL_ExtChrgSta_enum) -> VHAL_ExtChrgSta_enum/1
  [DT_CAN3_SG_BMS6] -> bus_selector14/1
  bus_selector14/1 -> HVBContactorSta/1(HVBContactorSta)  "<CAN3_HVBContactorSta>"
  HVBContactorSta/1(VHAL_HVBContactorSta_flg) -> VHAL_HVBContactorSta_flg/1
  [DT_CAN3_SG_BMS6] -> bus_selector15/1
  bus_selector15/1 -> HVBHVILErr/1(HVBHVILErr)  "<CAN3_HVBHVILErr>"
  HVBHVILErr/1(VHAL_HVBHVILErr_flg) -> VHAL_HVBHVILErr_flg/1
  [DT_CAN3_SG_BMS6] -> bus_selector16/1
  bus_selector16/1 -> HVBPreheatPrecoolSta/1(HVBPreheatPrecoolSta)  "<CAN3_HVBPreheatPrecoolSta>"
  HVBPreheatPrecoolSta/1(VHAL_HVBPreheatPrecoolSta_enum) -> VHAL_HVBPreheatPrecoolSta_enum/1
  [DT_CAN3_SG_BMS6] -> bus_selector17/1
  bus_selector17/1 -> HVBattReady4Pre/1(HVBattReady4Pre)  "<CAN3_HVBattReady4Pre>"
  HVBattReady4Pre/1(VHAL_HVBattReady4Pre_enum) -> VHAL_HVBattReady4Pre_enum/1
  [DT_CAN3_SG_BMS6] -> bus_selector18/1
  bus_selector18/1 -> HVILSta/1(HVILSta)  "<CAN3_HVILSta>"
  HVILSta/1(VHAL_HVILSta_flg) -> VHAL_HVILSta_flg/1
  [DT_CAN3_SG_BMS6] -> bus_selector19/1
  bus_selector19/1 -> V2LSta/1(V2LSta)  "<CAN3_V2LSta>"
  V2LSta/1(VHAL_V2LSta_enum) -> VHAL_V2LSta_enum/1

== system halin/HAL_IN/CAN3/BMS7 ==
  DT_CAN3_SG_BMS7 : Inport
  HVBattErr : Subsystem
  bus_selector : BusSelector  OutputSignals=CAN3_HVBattErr
  VHAL_HVBattErr_flg : Outport
  wires:
  DT_CAN3_SG_BMS7/1 -> [DT_CAN3_SG_BMS7]
  [DT_CAN3_SG_BMS7] -> bus_selector/1
  bus_selector/1 -> HVBattErr/1(HVBattErr)  "<CAN3_HVBattErr>"
  HVBattErr/1(VHAL_HVBattErr_flg) -> VHAL_HVBattErr_flg/1

== system halin/HAL_IN/CAN3/CCU1 ==
  DT_CAN3_SG_CCU1 : Inport
  0x35 : Constant  Value=0x35
  0xeb : Constant  Value=0xeb
  BitwiseAND{,1..11} (12 alike) : simulink/Logic and Bit Operations/Bitwise Operator  logicop=AND  UseBitMask=on  BitMask=0xFF  BitMaskRealWorld=Stored Integer
  BitwiseOR{,2,4..7} (6 alike) : simulink/Logic and Bit Operations/Bitwise Operator  logicop=OR  UseBitMask=off  BitMask=bin2dec('11011001')  BitMaskRealWorld=Stored Integer
  BitwiseOR1 : simulink/Logic and Bit Operations/Bitwise Operator  logicop=OR  UseBitMask=off  NumInputPorts=3  BitMask=bin2dec('11011001')  BitMaskRealWorld=Stored Integer
  BitwiseOR3 : simulink/Logic and Bit Operations/Bitwise Operator  logicop=OR  UseBitMask=off  NumInputPorts=3  BitMask=bin2dec('11011001')  BitMaskRealWorld=Stored Integer
  CSCCU1 : Subsystem
  DCDCAuxVolt : Subsystem
  DCDCInVoltInf : Subsystem
  DCDCPreCompleted : Subsystem
  DDM_CS&RC_Comparison : FVT_lib/hal/DDM_CS&RC_Comparison  MsgCycleTime=10
  Data Type Conversion{,1..11} (12 alike) : DataTypeConversion  OutDataTypeStr=uint8
  KHAL_CAN3CCU1E2E_flg : Constant  Value=KHAL_CAN3CCU1E2E_flg
  LeftShift : ArithShift  BitShiftDirection=Left
  LeftShift1 : ArithShift  BitShiftDirection=Left
  LeftShift2 : ArithShift  BitShiftNumber=4  BitShiftDirection=Left
  LeftShift3 : ArithShift  BitShiftNumber=6  BitShiftDirection=Left
  LeftShift4 : ArithShift  BitShiftNumber=2  BitShiftDirection=Left
  LeftShift5 : ArithShift  BitShiftDirection=Left
  MessageRollingCounter : FVT_lib/hal/MessageRollingCounter  CounterMAX=14  task_time_ms=5  msg_time_ms=10
  Mux : Mux  Inputs=7
  OBCDCCurrInf : Subsystem
  OBCDCVoltInf : Subsystem
  OBCPreCompleted : Subsystem
  OBCWakeup4Plugin : Subsystem
  RCCCU1 : Subsystem
  RightShift : ArithShift  BitShiftNumber=8
  RightShift1 : ArithShift
  RightShift2 : ArithShift  BitShiftNumber=8
  RightShift3 : ArithShift
  RightShift4 : ArithShift  BitShiftNumber=4
  RightShift5 : ArithShift  BitShiftNumber=-4
  bus_selector : BusSelector  OutputSignals=CAN3_CS_CCU1,CAN3_DCDCAuxVolt,CAN3_DCDCInVoltInf,CAN3_DCDCPreCompleted,CAN3_OBCDCCurrInf,CAN3_OBCDCVoltInf,CAN3_OBCPreCompleted,CAN3_OBCWakeup4Plugin,CAN3_RC_CCU1
  bus_selector1 : BusSelector  OutputSignals=CAN3_CS_CCU1
  bus_selector2 : BusSelector  OutputSignals=CAN3_DCDCAuxVolt
  bus_selector3 : BusSelector  OutputSignals=CAN3_DCDCInVoltInf
  bus_selector4 : BusSelector  OutputSignals=CAN3_DCDCPreCompleted
  bus_selector5 : BusSelector  OutputSignals=CAN3_OBCDCCurrInf
  bus_selector6 : BusSelector  OutputSignals=CAN3_OBCDCVoltInf
  bus_selector7 : BusSelector  OutputSignals=CAN3_OBCPreCompleted
  bus_selector8 : BusSelector  OutputSignals=CAN3_OBCWakeup4Plugin
  bus_selector9 : BusSelector  OutputSignals=CAN3_RC_CCU1
  VHAL_CCU1CSErr_flg : Outport
  VHAL_CCU1RCErr_flg : Outport  Port=2
  VHAL_CSCCU1_enum : Outport  Port=3
  VHAL_DCDCAuxVolt_V : Outport  Port=4
  VHAL_DCDCInVoltInf_V : Outport  Port=5
  VHAL_DCDCPreCompleted_enum : Outport  Port=6
  VHAL_OBCDCCurrInf_A : Outport  Port=7
  VHAL_OBCDCVoltInf_V : Outport  Port=8
  VHAL_OBCPreCompleted_enum : Outport  Port=9
  VHAL_OBCWakeup4Plugin_flg : Outport  Port=10
  VHAL_RCCCU1_enum : Outport  Port=11
  wires:
  DT_CAN3_SG_CCU1/1 -> [DT_CAN3_SG_CCU1]
  [DT_CAN3_SG_CCU1] -> bus_selector/1
  bus_selector/1 -> [CAN3_CS_CCU1]  "<CAN3_CS_CCU1>"
  [CAN3_CS_CCU1] -> LeftShift/1
  LeftShift/1 -> BitwiseAND/1
  BitwiseAND/1 -> [Byte_7_CAN3_CS_CCU1]
  bus_selector/2 -> [CAN3_DCDCAuxVolt]  "<CAN3_DCDCAuxVolt>"
  [CAN3_DCDCAuxVolt] -> LeftShift1/1
  LeftShift1/1 -> BitwiseAND1/1
  BitwiseAND1/1 -> [Byte_6_CAN3_DCDCAuxVolt]
  bus_selector/3 -> [CAN3_DCDCInVoltInf]  "<CAN3_DCDCInVoltInf>"
  [CAN3_DCDCInVoltInf] -> RightShift/1, RightShift1/1
  RightShift/1 -> BitwiseAND2/1
  BitwiseAND2/1 -> [Byte_3_CAN3_DCDCInVoltInf]
  RightShift1/1 -> BitwiseAND3/1
  BitwiseAND3/1 -> [Byte_4_CAN3_DCDCInVoltInf]
  bus_selector/4 -> [CAN3_DCDCPreCompleted]  "<CAN3_DCDCPreCompleted>"
  [CAN3_DCDCPreCompleted] -> LeftShift2/1
  LeftShift2/1 -> BitwiseAND4/1
  BitwiseAND4/1 -> [Byte_3_CAN3_DCDCPreCompleted]
  bus_selector/5 -> [CAN3_OBCDCCurrInf]  "<CAN3_OBCDCCurrInf>"
  [CAN3_OBCDCCurrInf] -> RightShift2/1, RightShift3/1
  RightShift2/1 -> BitwiseAND5/1
  BitwiseAND5/1 -> [Byte_1_CAN3_OBCDCCurrInf]
  RightShift3/1 -> BitwiseAND6/1
  BitwiseAND6/1 -> [Byte_2_CAN3_OBCDCCurrInf]
  bus_selector/6 -> [CAN3_OBCDCVoltInf]  "<CAN3_OBCDCVoltInf>"
  [CAN3_OBCDCVoltInf] -> RightShift4/1, RightShift5/1
  RightShift4/1 -> BitwiseAND7/1
  BitwiseAND7/1 -> [Byte_0_CAN3_OBCDCVoltInf]
  RightShift5/1 -> BitwiseAND8/1
  BitwiseAND8/1 -> [Byte_1_CAN3_OBCDCVoltInf]
  bus_selector/7 -> [CAN3_OBCPreCompleted]  "<CAN3_OBCPreCompleted>"
  [CAN3_OBCPreCompleted] -> LeftShift3/1
  LeftShift3/1 -> BitwiseAND9/1
  BitwiseAND9/1 -> [Byte_3_CAN3_OBCPreCompleted]
  bus_selector/8 -> [CAN3_OBCWakeup4Plugin]  "<CAN3_OBCWakeup4Plugin>"
  [CAN3_OBCWakeup4Plugin] -> LeftShift4/1
  LeftShift4/1 -> BitwiseAND10/1
  BitwiseAND10/1 -> [Byte_1_CAN3_OBCWakeup4Plugin]
  bus_selector/9 -> [CAN3_RC_CCU1]  "<CAN3_RC_CCU1>"
  [CAN3_RC_CCU1] -> LeftShift5/1
  LeftShift5/1 -> BitwiseAND11/1
  BitwiseAND11/1 -> [Byte_5_CAN3_RC_CCU1]
  Data Type Conversion/1 -> BitwiseOR/1
  [Byte_0_CAN3_OBCDCVoltInf] -> Data Type Conversion/1
  BitwiseOR/1 -> [Byte_0]
  Data Type Conversion1/1 -> BitwiseOR1/1
  [Byte_1_CAN3_OBCDCCurrInf] -> Data Type Conversion1/1
  Data Type Conversion2/1 -> BitwiseOR1/2
  [Byte_1_CAN3_OBCDCVoltInf] -> Data Type Conversion2/1
  Data Type Conversion3/1 -> BitwiseOR1/3
  [Byte_1_CAN3_OBCWakeup4Plugin] -> Data Type Conversion3/1
  BitwiseOR1/1 -> [Byte_1]
  Data Type Conversion4/1 -> BitwiseOR2/1
  [Byte_2_CAN3_OBCDCCurrInf] -> Data Type Conversion4/1
  BitwiseOR2/1 -> [Byte_2]
  Data Type Conversion5/1 -> BitwiseOR3/1
  [Byte_3_CAN3_DCDCInVoltInf] -> Data Type Conversion5/1
  Data Type Conversion6/1 -> BitwiseOR3/2
  [Byte_3_CAN3_DCDCPreCompleted] -> Data Type Conversion6/1
  Data Type Conversion7/1 -> BitwiseOR3/3
  [Byte_3_CAN3_OBCPreCompleted] -> Data Type Conversion7/1
  BitwiseOR3/1 -> [Byte_3]
  Data Type Conversion8/1 -> BitwiseOR4/1
  [Byte_4_CAN3_DCDCInVoltInf] -> Data Type Conversion8/1
  BitwiseOR4/1 -> [Byte_4]
  Data Type Conversion9/1 -> BitwiseOR5/1
  [Byte_5_CAN3_RC_CCU1] -> Data Type Conversion9/1
  BitwiseOR5/1 -> [Byte_5]
  Data Type Conversion10/1 -> BitwiseOR6/1
  [Byte_6_CAN3_DCDCAuxVolt] -> Data Type Conversion10/1
  BitwiseOR6/1 -> [Byte_6]
  Data Type Conversion11/1 -> BitwiseOR7/1
  [Byte_7_CAN3_CS_CCU1] -> Data Type Conversion11/1
  BitwiseOR7/1 -> [Byte_7]
  [Byte_0] -> Mux/1
  [Byte_1] -> Mux/2
  [Byte_2] -> Mux/3
  [Byte_3] -> Mux/4
  [Byte_4] -> Mux/5
  [Byte_5] -> Mux/6
  [Byte_6] -> Mux/7
  Mux/1 -> [VHAL_CAN3CCU1noCS_raw]
  KHAL_CAN3CCU1E2E_flg/1 -> DDM_CS&RC_Comparison/1
  0x35/1 -> DDM_CS&RC_Comparison/2
  0xeb/1 -> DDM_CS&RC_Comparison/3
  [VHAL_CAN3CCU1noCS_raw] -> DDM_CS&RC_Comparison/4
  [Byte_7] -> DDM_CS&RC_Comparison/5
  [RC_ECU] -> DDM_CS&RC_Comparison/6
  MessageRollingCounter/1 -> DDM_CS&RC_Comparison/7
  DDM_CS&RC_Comparison/1 -> VHAL_CCU1CSErr_flg/1
  DDM_CS&RC_Comparison/2 -> VHAL_CCU1RCErr_flg/1
  [DT_CAN3_SG_CCU1] -> bus_selector1/1
  bus_selector1/1 -> CSCCU1/1(CS_CCU1)  "<CAN3_CS_CCU1>"
  CSCCU1/1(VHAL_CSCCU1_enum) -> VHAL_CSCCU1_enum/1
  [DT_CAN3_SG_CCU1] -> bus_selector2/1
  bus_selector2/1 -> DCDCAuxVolt/1(DCDCAuxVolt)  "<CAN3_DCDCAuxVolt>"
  DCDCAuxVolt/1(VHAL_DCDCAuxVolt_V) -> VHAL_DCDCAuxVolt_V/1
  [DT_CAN3_SG_CCU1] -> bus_selector3/1
  bus_selector3/1 -> DCDCInVoltInf/1(DCDCInVoltInf)  "<CAN3_DCDCInVoltInf>"
  DCDCInVoltInf/1(VHAL_DCDCInVoltInf_V) -> VHAL_DCDCInVoltInf_V/1
  [DT_CAN3_SG_CCU1] -> bus_selector4/1
  bus_selector4/1 -> DCDCPreCompleted/1(DCDCPreCompleted)  "<CAN3_DCDCPreCompleted>"
  DCDCPreCompleted/1(VHAL_DCDCPreCompleted_enum) -> VHAL_DCDCPreCompleted_enum/1
  [DT_CAN3_SG_CCU1] -> bus_selector5/1
  bus_selector5/1 -> OBCDCCurrInf/1(OBCDCCurrInf)  "<CAN3_OBCDCCurrInf>"
  OBCDCCurrInf/1(VHAL_OBCDCCurrInf_A) -> VHAL_OBCDCCurrInf_A/1
  [DT_CAN3_SG_CCU1] -> bus_selector6/1
  bus_selector6/1 -> OBCDCVoltInf/1(OBCDCVoltInf)  "<CAN3_OBCDCVoltInf>"
  OBCDCVoltInf/1(VHAL_OBCDCVoltInf_V) -> VHAL_OBCDCVoltInf_V/1
  [DT_CAN3_SG_CCU1] -> bus_selector7/1
  bus_selector7/1 -> OBCPreCompleted/1(OBCPreCompleted)  "<CAN3_OBCPreCompleted>"
  OBCPreCompleted/1(VHAL_OBCPreCompleted_enum) -> VHAL_OBCPreCompleted_enum/1
  [DT_CAN3_SG_CCU1] -> bus_selector8/1
  bus_selector8/1 -> OBCWakeup4Plugin/1(OBCWakeup4Plugin)  "<CAN3_OBCWakeup4Plugin>"
  OBCWakeup4Plugin/1(VHAL_OBCWakeup4Plugin_flg) -> VHAL_OBCWakeup4Plugin_flg/1
  [DT_CAN3_SG_CCU1] -> bus_selector9/1
  bus_selector9/1 -> RCCCU1/1(RC_CCU1)  "<CAN3_RC_CCU1>"
  RCCCU1/1(VHAL_RCCCU1_enum) -> VHAL_RCCCU1_enum/1, [RC_ECU]

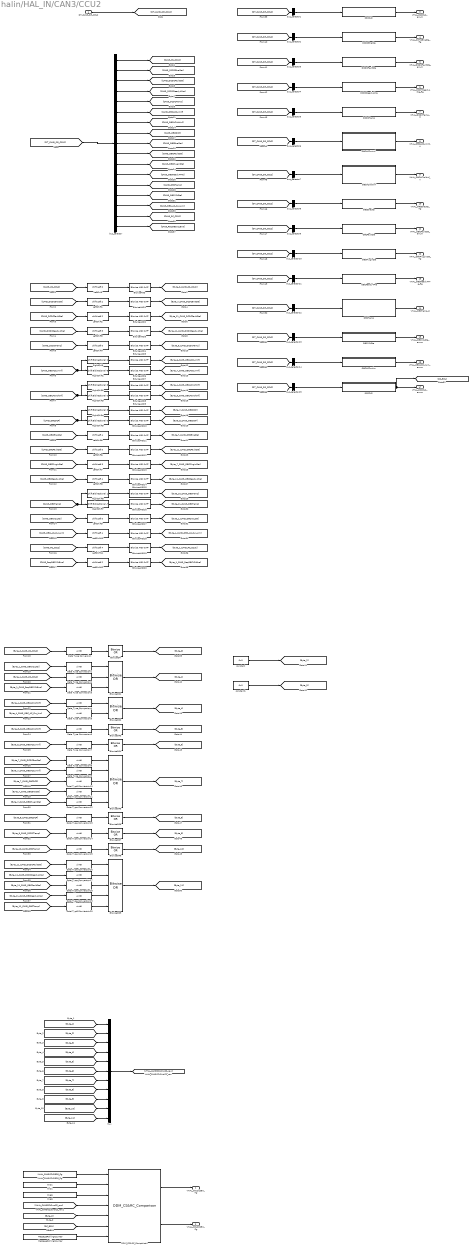
== system halin/HAL_IN/CAN3/CCU2 ==
  DT_CAN3_SG_CCU2 : Inport
  0x21 : Constant  Value=0x21
  0xe6 : Constant  Value=0xe6
  BitwiseAND{,1..20} (21 alike) : simulink/Logic and Bit Operations/Bitwise Operator  logicop=AND  UseBitMask=on  BitMask=0xFF  BitMaskRealWorld=Stored Integer
  BitwiseOR{,3..4,6..8} (6 alike) : simulink/Logic and Bit Operations/Bitwise Operator  logicop=OR  UseBitMask=off  BitMask=bin2dec('11011001')  BitMaskRealWorld=Stored Integer
  BitwiseOR1 : simulink/Logic and Bit Operations/Bitwise Operator  logicop=OR  UseBitMask=off  NumInputPorts=3  BitMask=bin2dec('11011001')  BitMaskRealWorld=Stored Integer
  BitwiseOR2 : simulink/Logic and Bit Operations/Bitwise Operator  logicop=OR  UseBitMask=off  NumInputPorts=2  BitMask=bin2dec('11011001')  BitMaskRealWorld=Stored Integer
  BitwiseOR5 : simulink/Logic and Bit Operations/Bitwise Operator  logicop=OR  UseBitMask=off  NumInputPorts=5  BitMask=bin2dec('11011001')  BitMaskRealWorld=Stored Integer
  BitwiseOR9 : simulink/Logic and Bit Operations/Bitwise Operator  logicop=OR  UseBitMask=off  NumInputPorts=5  BitMask=bin2dec('11011001')  BitMaskRealWorld=Stored Integer
  CSCCU2 : Subsystem
  DCDCEnaSta : Subsystem
  DCDCFaultSta : Subsystem
  DCDCReady4Pre : Subsystem
  DCDCTemp : Subsystem
  DDM_CS&RC_Comparison : FVT_lib/hal/DDM_CS&RC_Comparison  MsgCycleTime=100
  Data Type Conversion{,1..20} (21 alike) : DataTypeConversion  OutDataTypeStr=uint8
  KHAL_CAN3CCU2E2E_flg : Constant  Value=KHAL_CAN3CCU2E2E_flg
  LeftShift{,4,6,9} (4 alike) : ArithShift  BitShiftDirection=Left
  LeftShift1 : ArithShift  BitShiftNumber=2  BitShiftDirection=Left
  LeftShift{5,8,10..11} (4 alike) : ArithShift  BitShiftNumber=4  BitShiftDirection=Left
  LeftShift12 : ArithShift  BitShiftNumber=2  BitShiftDirection=Left
  LeftShift2 : ArithShift  BitShiftNumber=2  BitShiftDirection=Left
  LeftShift3 : ArithShift  BitShiftNumber=5  BitShiftDirection=Left
  LeftShift7 : ArithShift  BitShiftNumber=3  BitShiftDirection=Left
  MessageRollingCounter : FVT_lib/hal/MessageRollingCounter  CounterMAX=14  task_time_ms=5  msg_time_ms=100
  Mux : Mux  Inputs=11
  OBCACCurLim : Subsystem
  OBCACCurrInf : Subsystem
  OBCACVoltInf : Subsystem
  OBCEnaSta : Subsystem
  OBCFaultSta : Subsystem
  OBCPluginSta : Subsystem
  OBCReady4Pre : Subsystem
  OBCTemp : Subsystem
  OBCV2LSta : Subsystem
  RCCCU2 : Subsystem
  RightShift : ArithShift  BitShiftNumber=2
  RightShift1 : ArithShift  BitShiftNumber=-6
  RightShift2 : ArithShift  BitShiftNumber=8
  RightShift3 : ArithShift
  RightShift4 : ArithShift  BitShiftNumber=8
  RightShift5 : ArithShift
  RightShift6 : ArithShift  BitShiftNumber=1
  RightShift7 : ArithShift  BitShiftNumber=-7
  bus_selector : BusSelector  OutputSignals=CAN3_CS_CCU2,CAN3_DCDCEnaSta,CAN3_DCDCFaultSta,CAN3_DCDCReady4Pre,CAN3_DCDCTemp,CAN3_OBCACCurrInf,CAN3_OBCACVoltInf,CAN3_OBCDCP,CAN3_OBCEnaSta,CAN3_OBCFaultSta,CAN3_OBCPluginSta,CAN3_OBCReady4Pre,CAN3_OBCTemp,CAN3_OBCV2LSta,CAN3_OBC_AC_Cur_Lim,CAN3_RC_CCU2,CAN3_ReqOBCV2LEna
  bus_selector1 : BusSelector  OutputSignals=CAN3_CS_CCU2
  bus_selector10 : BusSelector  OutputSignals=CAN3_OBCPluginSta
  bus_selector11 : BusSelector  OutputSignals=CAN3_OBCReady4Pre
  bus_selector12 : BusSelector  OutputSignals=CAN3_OBCTemp
  bus_selector13 : BusSelector  OutputSignals=CAN3_OBCV2LSta
  bus_selector14 : BusSelector  OutputSignals=CAN3_OBC_AC_Cur_Lim
  bus_selector15 : BusSelector  OutputSignals=CAN3_RC_CCU2
  bus_selector2 : BusSelector  OutputSignals=CAN3_DCDCEnaSta
  bus_selector3 : BusSelector  OutputSignals=CAN3_DCDCFaultSta
  bus_selector4 : BusSelector  OutputSignals=CAN3_DCDCReady4Pre
  bus_selector5 : BusSelector  OutputSignals=CAN3_DCDCTemp
  bus_selector6 : BusSelector  OutputSignals=CAN3_OBCACCurrInf
  bus_selector7 : BusSelector  OutputSignals=CAN3_OBCACVoltInf
  bus_selector8 : BusSelector  OutputSignals=CAN3_OBCEnaSta
  bus_selector9 : BusSelector  OutputSignals=CAN3_OBCFaultSta
  constant : Constant  Value=0x0  OutDataTypeStr=uint8
  constant1 : Constant  Value=0x0  OutDataTypeStr=uint8
  VHAL_CCU2CSErr_flg : Outport
  VHAL_CCU2RCErr_flg : Outport  Port=2
  VHAL_CSCCU2_enum : Outport  Port=3
  VHAL_DCDCEnaSta_flg : Outport  Port=4
  VHAL_DCDCFaultSta_enum : Outport  Port=5
  VHAL_DCDCReady4Pre_flg : Outport  Port=6
  VHAL_DCDCTemp_C : Outport  Port=7
  VHAL_OBCACCurrInf_A : Outport  Port=8
  VHAL_OBCACVoltInf_V : Outport  Port=9
  VHAL_OBCEnaSta_flg : Outport  Port=10
  VHAL_OBCFaultSta_enum : Outport  Port=11
  VHAL_OBCPluginSta_flg : Outport  Port=12
  VHAL_OBCReady4Pre_flg : Outport  Port=13
  VHAL_OBCTemp_C : Outport  Port=14
  VHAL_OBCV2LSta_enum : Outport  Port=15
  VHAL_OBCACCurLim_enum : Outport  Port=16
  VHAL_RCCCU2_enum : Outport  Port=17
  wires:
  DT_CAN3_SG_CCU2/1 -> [DT_CAN3_SG_CCU2]
  [DT_CAN3_SG_CCU2] -> bus_selector/1
  bus_selector/1 -> [CAN3_CS_CCU2]  "<CAN3_CS_CCU2>"
  [CAN3_CS_CCU2] -> LeftShift/1
  LeftShift/1 -> BitwiseAND/1
  BitwiseAND/1 -> [Byte_0_CAN3_CS_CCU2]
  bus_selector/2 -> [CAN3_DCDCEnaSta]  "<CAN3_DCDCEnaSta>"
  [CAN3_DCDCEnaSta] -> LeftShift1/1
  LeftShift1/1 -> BitwiseAND1/1
  BitwiseAND1/1 -> [Byte_7_CAN3_DCDCEnaSta]
  bus_selector/3 -> [CAN3_DCDCFaultSta]  "<CAN3_DCDCFaultSta>"
  [CAN3_DCDCFaultSta] -> LeftShift2/1
  LeftShift2/1 -> BitwiseAND2/1
  BitwiseAND2/1 -> [Byte_11_CAN3_DCDCFaultSta]
  bus_selector/4 -> [CAN3_DCDCReady4Pre]  "<CAN3_DCDCReady4Pre>"
  [CAN3_DCDCReady4Pre] -> LeftShift3/1
  LeftShift3/1 -> BitwiseAND3/1
  BitwiseAND3/1 -> [Byte_11_CAN3_DCDCReady4Pre]
  bus_selector/5 -> [CAN3_DCDCTemp]  "<CAN3_DCDCTemp>"
  [CAN3_DCDCTemp] -> LeftShift4/1
  LeftShift4/1 -> BitwiseAND4/1
  BitwiseAND4/1 -> [Byte_9_CAN3_DCDCTemp]
  bus_selector/6 -> [CAN3_OBCACCurrInf]  "<CAN3_OBCACCurrInf>"
  [CAN3_OBCACCurrInf] -> RightShift/1, RightShift1/1
  RightShift/1 -> BitwiseAND5/1
  BitwiseAND5/1 -> [Byte_6_CAN3_OBCACCurrInf]
  RightShift1/1 -> BitwiseAND6/1
  BitwiseAND6/1 -> [Byte_7_CAN3_OBCACCurrInf]
  bus_selector/7 -> [CAN3_OBCACVoltInf]  "<CAN3_OBCACVoltInf>"
  [CAN3_OBCACVoltInf] -> RightShift2/1, RightShift3/1
  RightShift2/1 -> BitwiseAND7/1
  BitwiseAND7/1 -> [Byte_4_CAN3_OBCACVoltInf]
  RightShift3/1 -> BitwiseAND8/1
  BitwiseAND8/1 -> [Byte_5_CAN3_OBCACVoltInf]
  bus_selector/8 -> [CAN3_OBCDCP]  "<CAN3_OBCDCP>"
  [CAN3_OBCDCP] -> RightShift4/1, RightShift5/1
  RightShift4/1 -> BitwiseAND9/1
  BitwiseAND9/1 -> [Byte_7_CAN3_OBCDCP]
  RightShift5/1 -> BitwiseAND10/1
  BitwiseAND10/1 -> [Byte_8_CAN3_OBCDCP]
  bus_selector/9 -> [CAN3_OBCEnaSta]  "<CAN3_OBCEnaSta>"
  [CAN3_OBCEnaSta] -> LeftShift5/1
  LeftShift5/1 -> BitwiseAND11/1
  BitwiseAND11/1 -> [Byte_7_CAN3_OBCEnaSta]
  bus_selector/10 -> [CAN3_OBCFaultSta]  "<CAN3_OBCFaultSta>"
  [CAN3_OBCFaultSta] -> LeftShift6/1
  LeftShift6/1 -> BitwiseAND12/1
  BitwiseAND12/1 -> [Byte_11_CAN3_OBCFaultSta]
  bus_selector/11 -> [CAN3_OBCPluginSta]  "<CAN3_OBCPluginSta>"
  [CAN3_OBCPluginSta] -> LeftShift7/1
  LeftShift7/1 -> BitwiseAND13/1
  BitwiseAND13/1 -> [Byte_7_CAN3_OBCPluginSta]
  bus_selector/12 -> [CAN3_OBCReady4Pre]  "<CAN3_OBCReady4Pre>"
  [CAN3_OBCReady4Pre] -> LeftShift8/1
  LeftShift8/1 -> BitwiseAND14/1
  BitwiseAND14/1 -> [Byte_11_CAN3_OBCReady4Pre]
  bus_selector/13 -> [CAN3_OBCTemp]  "<CAN3_OBCTemp>"
  [CAN3_OBCTemp] -> RightShift6/1, RightShift7/1
  RightShift6/1 -> BitwiseAND15/1
  BitwiseAND15/1 -> [Byte_10_CAN3_OBCTemp]
  RightShift7/1 -> BitwiseAND16/1
  BitwiseAND16/1 -> [Byte_11_CAN3_OBCTemp]
  bus_selector/14 -> [CAN3_OBCV2LSta]  "<CAN3_OBCV2LSta>"
  [CAN3_OBCV2LSta] -> LeftShift9/1
  LeftShift9/1 -> BitwiseAND17/1
  BitwiseAND17/1 -> [Byte_1_CAN3_OBCV2LSta]
  bus_selector/15 -> [CAN3_OBC_AC_Cur_Lim]  "<CAN3_OBC_AC_Cur_Lim>"
  [CAN3_OBC_AC_Cur_Lim] -> LeftShift10/1
  LeftShift10/1 -> BitwiseAND18/1
  BitwiseAND18/1 -> [Byte_4_CAN3_OBC_AC_Cur_Lim]
  bus_selector/16 -> [CAN3_RC_CCU2]  "<CAN3_RC_CCU2>"
  [CAN3_RC_CCU2] -> LeftShift11/1
  LeftShift11/1 -> BitwiseAND19/1
  BitwiseAND19/1 -> [Byte_1_CAN3_RC_CCU2]
  bus_selector/17 -> [CAN3_ReqOBCV2LEna]  "<CAN3_ReqOBCV2LEna>"
  [CAN3_ReqOBCV2LEna] -> LeftShift12/1
  LeftShift12/1 -> BitwiseAND20/1
  BitwiseAND20/1 -> [Byte_1_CAN3_ReqOBCV2LEna]
  Data Type Conversion/1 -> BitwiseOR/1
  [Byte_0_CAN3_CS_CCU2] -> Data Type Conversion/1
  BitwiseOR/1 -> [Byte_0]
  Data Type Conversion1/1 -> BitwiseOR1/1
  [Byte_1_CAN3_OBCV2LSta] -> Data Type Conversion1/1
  Data Type Conversion2/1 -> BitwiseOR1/2
  [Byte_1_CAN3_RC_CCU2] -> Data Type Conversion2/1
  Data Type Conversion3/1 -> BitwiseOR1/3
  [Byte_1_CAN3_ReqOBCV2LEna] -> Data Type Conversion3/1
  BitwiseOR1/1 -> [Byte_1]
  constant/1 -> [Byte_2]
  constant1/1 -> [Byte_3]
  Data Type Conversion4/1 -> BitwiseOR2/1
  [Byte_4_CAN3_OBCACVoltInf] -> Data Type Conversion4/1
  Data Type Conversion5/1 -> BitwiseOR2/2
  [Byte_4_CAN3_OBC_AC_Cur_Lim] -> Data Type Conversion5/1
  BitwiseOR2/1 -> [Byte_4]
  Data Type Conversion6/1 -> BitwiseOR3/1
  [Byte_5_CAN3_OBCACVoltInf] -> Data Type Conversion6/1
  BitwiseOR3/1 -> [Byte_5]
  Data Type Conversion7/1 -> BitwiseOR4/1
  [Byte_6_CAN3_OBCACCurrInf] -> Data Type Conversion7/1
  BitwiseOR4/1 -> [Byte_6]
  Data Type Conversion8/1 -> BitwiseOR5/1
  [Byte_7_CAN3_DCDCEnaSta] -> Data Type Conversion8/1
  Data Type Conversion9/1 -> BitwiseOR5/2
  [Byte_7_CAN3_OBCACCurrInf] -> Data Type Conversion9/1
  Data Type Conversion10/1 -> BitwiseOR5/3
  [Byte_7_CAN3_OBCDCP] -> Data Type Conversion10/1
  Data Type Conversion11/1 -> BitwiseOR5/4
  [Byte_7_CAN3_OBCEnaSta] -> Data Type Conversion11/1
  Data Type Conversion12/1 -> BitwiseOR5/5
  [Byte_7_CAN3_OBCPluginSta] -> Data Type Conversion12/1
  BitwiseOR5/1 -> [Byte_7]
  Data Type Conversion13/1 -> BitwiseOR6/1
  [Byte_8_CAN3_OBCDCP] -> Data Type Conversion13/1
  BitwiseOR6/1 -> [Byte_8]
  Data Type Conversion14/1 -> BitwiseOR7/1
  [Byte_9_CAN3_DCDCTemp] -> Data Type Conversion14/1
  BitwiseOR7/1 -> [Byte_9]
  Data Type Conversion15/1 -> BitwiseOR8/1
  [Byte_10_CAN3_OBCTemp] -> Data Type Conversion15/1
  BitwiseOR8/1 -> [Byte_10]
  Data Type Conversion16/1 -> BitwiseOR9/1
  [Byte_11_CAN3_DCDCFaultSta] -> Data Type Conversion16/1
  Data Type Conversion17/1 -> BitwiseOR9/2
  [Byte_11_CAN3_DCDCReady4Pre] -> Data Type Conversion17/1
  Data Type Conversion18/1 -> BitwiseOR9/3
  [Byte_11_CAN3_OBCFaultSta] -> Data Type Conversion18/1
  Data Type Conversion19/1 -> BitwiseOR9/4
  [Byte_11_CAN3_OBCReady4Pre] -> Data Type Conversion19/1
  Data Type Conversion20/1 -> BitwiseOR9/5
  [Byte_11_CAN3_OBCTemp] -> Data Type Conversion20/1
  BitwiseOR9/1 -> [Byte_11]
  [Byte_1] -> Mux/1
  [Byte_2] -> Mux/2
  [Byte_3] -> Mux/3
  [Byte_4] -> Mux/4
  [Byte_5] -> Mux/5
  [Byte_6] -> Mux/6
  [Byte_7] -> Mux/7
  [Byte_8] -> Mux/8
  [Byte_9] -> Mux/9
  [Byte_10] -> Mux/10
  [Byte_11] -> Mux/11
  Mux/1 -> [VHAL_CAN3CCU2noCS_raw]
  KHAL_CAN3CCU2E2E_flg/1 -> DDM_CS&RC_Comparison/1
  0x21/1 -> DDM_CS&RC_Comparison/2
  0xe6/1 -> DDM_CS&RC_Comparison/3
  [VHAL_CAN3CCU2noCS_raw] -> DDM_CS&RC_Comparison/4
  [Byte_0] -> DDM_CS&RC_Comparison/5
  [RC_ECU] -> DDM_CS&RC_Comparison/6
  MessageRollingCounter/1 -> DDM_CS&RC_Comparison/7
  DDM_CS&RC_Comparison/1 -> VHAL_CCU2CSErr_flg/1
  DDM_CS&RC_Comparison/2 -> VHAL_CCU2RCErr_flg/1
  [DT_CAN3_SG_CCU2] -> bus_selector1/1
  bus_selector1/1 -> CSCCU2/1(CS_CCU2)  "<CAN3_CS_CCU2>"
  CSCCU2/1(VHAL_CSCCU2_enum) -> VHAL_CSCCU2_enum/1
  [DT_CAN3_SG_CCU2] -> bus_selector2/1
  bus_selector2/1 -> DCDCEnaSta/1(DCDCEnaSta)  "<CAN3_DCDCEnaSta>"
  DCDCEnaSta/1(VHAL_DCDCEnaSta_flg) -> VHAL_DCDCEnaSta_flg/1
  [DT_CAN3_SG_CCU2] -> bus_selector3/1
  bus_selector3/1 -> DCDCFaultSta/1(DCDCFaultSta)  "<CAN3_DCDCFaultSta>"
  DCDCFaultSta/1(VHAL_DCDCFaultSta_enum) -> VHAL_DCDCFaultSta_enum/1
  [DT_CAN3_SG_CCU2] -> bus_selector4/1
  bus_selector4/1 -> DCDCReady4Pre/1(DCDCReady4Pre)  "<CAN3_DCDCReady4Pre>"
  DCDCReady4Pre/1(VHAL_DCDCReady4Pre_flg) -> VHAL_DCDCReady4Pre_flg/1
  [DT_CAN3_SG_CCU2] -> bus_selector5/1
  bus_selector5/1 -> DCDCTemp/1(DCDCTemp)  "<CAN3_DCDCTemp>"
  DCDCTemp/1(VHAL_DCDCTemp_C) -> VHAL_DCDCTemp_C/1
  [DT_CAN3_SG_CCU2] -> bus_selector6/1
  bus_selector6/1 -> OBCACCurrInf/1(OBCACCurrInf)  "<CAN3_OBCACCurrInf>"
  OBCACCurrInf/1(VHAL_OBCACCurrInf_A) -> VHAL_OBCACCurrInf_A/1
  [DT_CAN3_SG_CCU2] -> bus_selector7/1
  bus_selector7/1 -> OBCACVoltInf/1(OBCACVoltInf)  "<CAN3_OBCACVoltInf>"
  OBCACVoltInf/1(VHAL_OBCACVoltInf_V) -> VHAL_OBCACVoltInf_V/1
  [DT_CAN3_SG_CCU2] -> bus_selector8/1
  bus_selector8/1 -> OBCEnaSta/1(OBCEnaSta)  "<CAN3_OBCEnaSta>"
  OBCEnaSta/1(VHAL_OBCEnaSta_flg) -> VHAL_OBCEnaSta_flg/1
  [DT_CAN3_SG_CCU2] -> bus_selector9/1
  bus_selector9/1 -> OBCFaultSta/1(OBCFaultSta)  "<CAN3_OBCFaultSta>"
  OBCFaultSta/1(VHAL_OBCFaultSta_enum) -> VHAL_OBCFaultSta_enum/1
  [DT_CAN3_SG_CCU2] -> bus_selector10/1
  bus_selector10/1 -> OBCPluginSta/1(OBCPluginSta)  "<CAN3_OBCPluginSta>"
  OBCPluginSta/1(VHAL_OBCPluginSta_flg) -> VHAL_OBCPluginSta_flg/1
  [DT_CAN3_SG_CCU2] -> bus_selector11/1
  bus_selector11/1 -> OBCReady4Pre/1(OBCReady4Pre)  "<CAN3_OBCReady4Pre>"
  OBCReady4Pre/1(VHAL_OBCReady4Pre_flg) -> VHAL_OBCReady4Pre_flg/1
  [DT_CAN3_SG_CCU2] -> bus_selector12/1
  bus_selector12/1 -> OBCTemp/1(OBCTemp)  "<CAN3_OBCTemp>"
  OBCTemp/1(VHAL_OBCTemp_C) -> VHAL_OBCTemp_C/1
  [DT_CAN3_SG_CCU2] -> bus_selector13/1
  bus_selector13/1 -> OBCV2LSta/1(OBCV2LSta)  "<CAN3_OBCV2LSta>"
  OBCV2LSta/1(VHAL_OBCV2LSta_enum) -> VHAL_OBCV2LSta_enum/1
  [DT_CAN3_SG_CCU2] -> bus_selector14/1
  bus_selector14/1 -> OBCACCurLim/1(OBC_AC_Cur_Lim)  "<CAN3_OBC_AC_Cur_Lim>"
  OBCACCurLim/1(VHAL_OBCACCurLim_enum) -> VHAL_OBCACCurLim_enum/1
  [DT_CAN3_SG_CCU2] -> bus_selector15/1
  bus_selector15/1 -> RCCCU2/1(RC_CCU2)  "<CAN3_RC_CCU2>"
  RCCCU2/1(VHAL_RCCCU2_enum) -> VHAL_RCCCU2_enum/1, [RC_ECU]

== system halin/HAL_IN/CAN3/CCU4 ==
  DT_CAN3_SG_CCU4 : Inport
  DCDCAuxCur : Subsystem
  DCDCHVCur : Subsystem
  bus_selector : BusSelector  OutputSignals=CAN3_DCDCAuxCur
  bus_selector1 : BusSelector  OutputSignals=CAN3_DCDCHVCur
  VHAL_DCDCAuxCur_A : Outport
  VHAL_DCDCHVCur_A : Outport  Port=2
  wires:
  DT_CAN3_SG_CCU4/1 -> [DT_CAN3_SG_CCU4]
  [DT_CAN3_SG_CCU4] -> bus_selector/1
  bus_selector/1 -> DCDCAuxCur/1(DCDCAuxCur)  "<CAN3_DCDCAuxCur>"
  DCDCAuxCur/1(VHAL_DCDCAuxCur_A) -> VHAL_DCDCAuxCur_A/1
  [DT_CAN3_SG_CCU4] -> bus_selector1/1
  bus_selector1/1 -> DCDCHVCur/1(DCDCHVCur)  "<CAN3_DCDCHVCur>"
  DCDCHVCur/1(VHAL_DCDCHVCur_A) -> VHAL_DCDCHVCur_A/1
